simulink model "SimulinkLabPartTwo"  (R2024b)
settings: Solver=VariableStepAuto  StartTime=0.0  StopTime=10.0  RelTol=1e-3
libraries: simulink x31
settings Model: Creator=ferbe  LastModifiedBy=ferbe

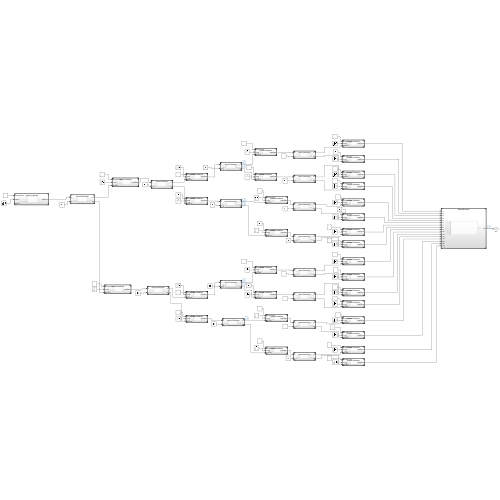
[thumbnail: Simulink's stored preview of the top-level diagram]
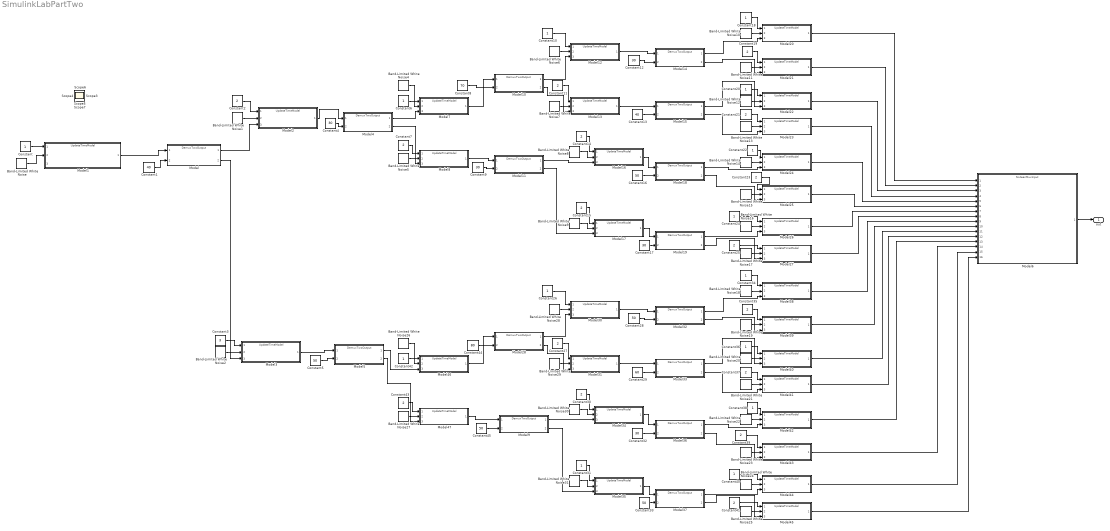
== system SimulinkLabPartTwo ==
  Band-Limited White Noise{,1..2,4..31} (31 alike) : simulink/Sources/Band-Limited White Noise  Cov=[0.01]  Ts=0.1  seed=[23341]
  Constant{,6,10,18,20,22,24,26,31,34,36,38,40,42} (14 alike) : Constant
  Constant1 : Constant  Value=40
  Constant{2,7,11,14..15,19,21,23,25,27,30,35,37,39,41,43} (16 alike) : Constant  Value=2
  Constant{4,9,12,17,32} (5 alike) : Constant  Value=30
  Constant13 : Constant  Value=40
  Constant{5,16,28,33,45} (5 alike) : Constant  Value=50
  Constant29 : Constant  Value=60
  Constant3 : Constant  Value=3
  Constant44 : Constant  Value=80
  Constant8 : Constant  Value=70
  Model{,4..5,9..11,14..15,18..19,28,32..33,36..37} (15 alike) : ModelReference  ModelNameDialog=DemuxTwoOutput.slx  SimulationMode=Normal  ModelReferenceVersion=1.22
  Model{1..3,7..8,12..13,16..17,20..27,30..31,34..35,38..47} (31 alike) : ModelReference  ModelNameDialog=UpdateTimeModel.slx  SimulationMode=Normal  ModelReferenceVersion=5.5
  Model6 : ModelReference  ModelNameDialog=SixteenMuxInput.slx  SimulationMode=Normal  ModelReferenceVersion=1.1
  out : Outport
  Scope{,1..7} (8 alike) : Scope
  wires:
  Constant/1 -> Model1/1
  Band-Limited White Noise/1 -> Model1/2
  Model1/1 -> Model/1
  Constant1/1 -> Model/2
  Model/1 -> Model2/3
  Band-Limited White Noise1/1 -> Model2/2
  Constant2/1 -> Model2/1
  Band-Limited White Noise2/1 -> Model3/2
  Constant3/1 -> Model3/1
  Model/2 -> Model3/3
  Model2/1 -> Model4/1
  Constant4/1 -> Model4/2
  Constant5/1 -> Model5/2
  Model3/1 -> Model5/1
  Model4/1 -> Model7/3
  Constant6/1 -> Model7/1
  Band-Limited White Noise4/1 -> Model7/2
  Band-Limited White Noise5/1 -> Model8/2
  Model4/2 -> Model8/3
  Constant7/1 -> Model8/1
  Model7/1 -> Model10/1
  Constant8/1 -> Model10/2
  Model8/1 -> Model11/1
  Constant9/1 -> Model11/2
  Band-Limited White Noise6/1 -> Model12/2
  Model10/1 -> Model12/3
  Constant10/1 -> Model12/1
  Model10/2 -> Model13/3
  Band-Limited White Noise7/1 -> Model13/2
  Constant11/1 -> Model13/1
  Model12/1 -> Model14/1
  Constant12/1 -> Model14/2
  Model13/1 -> Model15/1
  Constant13/1 -> Model15/2
  Band-Limited White Noise8/1 -> Model16/2
  Model11/1 -> Model16/3
  Constant14/1 -> Model16/1
  Band-Limited White Noise9/1 -> Model17/2
  Constant15/1 -> Model17/1
  Model11/2 -> Model17/3
  Model16/1 -> Model18/1
  Constant16/1 -> Model18/2
  Model17/1 -> Model19/1
  Constant17/1 -> Model19/2
  Band-Limited White Noise10/1 -> Model20/2
  Model14/1 -> Model20/3
  Constant18/1 -> Model20/1
  Band-Limited White Noise11/1 -> Model21/2
  Model14/2 -> Model21/3
  Constant19/1 -> Model21/1
  Band-Limited White Noise12/1 -> Model22/2
  Model15/1 -> Model22/3
  Constant20/1 -> Model22/1
  Constant21/1 -> Model23/1
  Model15/2 -> Model23/3
  Band-Limited White Noise13/1 -> Model23/2
  Constant22/1 -> Model24/1
  Model18/1 -> Model24/3
  Band-Limited White Noise14/1 -> Model24/2
  Constant23/1 -> Model25/1
  Model18/2 -> Model25/3
  Band-Limited White Noise15/1 -> Model25/2
  Constant24/1 -> Model26/1
  Model19/1 -> Model26/3
  Band-Limited White Noise16/1 -> Model26/2
  Constant25/1 -> Model27/1
  Model19/2 -> Model27/3
  Band-Limited White Noise17/1 -> Model27/2
  Band-Limited White Noise30/1 -> Model34/2
  Model32/1 -> Model38/3
  Model37/1 -> Model44/3
  Model35/1 -> Model37/1
  Constant32/1 -> Model36/2
  Band-Limited White Noise26/1 -> Model46/2
  Constant42/1 -> Model46/1
  Model28/1 -> Model30/3
  Band-Limited White Noise23/1 -> Model43/2
  Constant36/1 -> Model40/1
  Model32/2 -> Model39/3
  Constant28/1 -> Model32/2
  Constant43/1 -> Model47/1
  Constant27/1 -> Model31/1
  Band-Limited White Noise29/1 -> Model31/2
  Constant30/1 -> Model34/1
  Band-Limited White Noise28/1 -> Model30/2
  Constant35/1 -> Model39/1
  Band-Limited White Noise31/1 -> Model35/2
  Model34/1 -> Model36/1
  Constant34/1 -> Model38/1
  Constant26/1 -> Model30/1
  Model30/1 -> Model32/1
  Constant29/1 -> Model33/2
  Band-Limited White Noise27/1 -> Model47/2
  Constant44/1 -> Model28/2
  Band-Limited White Noise25/1 -> Model45/2
  Model31/1 -> Model33/1
  Model36/1 -> Model42/3
  Band-Limited White Noise24/1 -> Model44/2
  Band-Limited White Noise18/1 -> Model38/2
  Model33/1 -> Model40/3
  Constant38/1 -> Model42/1
  Constant41/1 -> Model45/1
  Model28/2 -> Model31/3
  Model33/2 -> Model41/3
  Band-Limited White Noise21/1 -> Model41/2
  Constant33/1 -> Model37/2
  Model46/1 -> Model28/1
  Constant40/1 -> Model44/1
  Model36/2 -> Model43/3
  Constant39/1 -> Model43/1
  Constant37/1 -> Model41/1
  Constant31/1 -> Model35/1
  Band-Limited White Noise20/1 -> Model40/2
  Model37/2 -> Model45/3
  Band-Limited White Noise22/1 -> Model42/2
  Band-Limited White Noise19/1 -> Model39/2
  Model5/1 -> Model46/3
  Model5/2 -> Model47/3
  Model20/1 -> Model6/1
  Model21/1 -> Model6/2
  Model22/1 -> Model6/3
  Model23/1 -> Model6/4
  Model24/1 -> Model6/5
  Model25/1 -> Model6/6
  Model26/1 -> Model6/7
  Model27/1 -> Model6/8
  Model38/1 -> Model6/9
  Model39/1 -> Model6/10
  Model40/1 -> Model6/11
  Model41/1 -> Model6/12
  Model42/1 -> Model6/13
  Model43/1 -> Model6/14
  Model44/1 -> Model6/15
  Model45/1 -> Model6/16
  Model6/1 -> out/1
  Model9/1 -> Model34/3
  Model47/1 -> Model9/1
  Constant45/1 -> Model9/2
  Model9/2 -> Model35/3
